simulink model "Model_SinglePhase_TwoArm"  (R2022a)
settings: Solver=VariableStepAuto  StartTime=0.0  StopTime=10.0  RelTol=1e-3
libraries: fl_lib x15
settings Model: Creator=chack  LastModifiedBy=chack

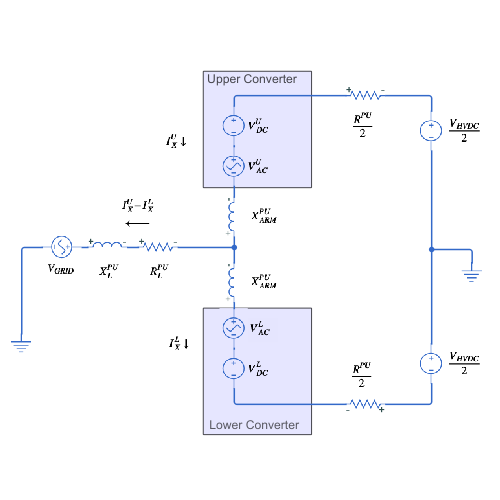
[thumbnail: Simulink's stored preview of the top-level diagram]
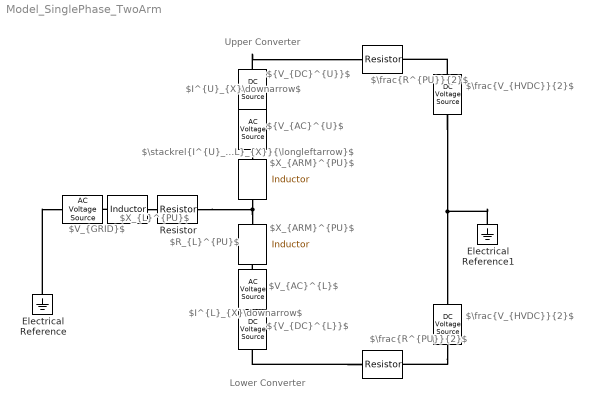
== system Model_SinglePhase_TwoArm ==
  note: $I^{U}_{X}\downarrow$
  note: Lower Converter
  note: Upper Converter
  note: ${V_{DC}^{U}}$
  note: $V_{GRID}$
  note: $R_{L}^{PU}$
  note: $X_{L}^{PU}$
  note: $\frac{V_{HVDC}}{2}$
  note: $\frac{V_{HVDC}}{2}$
  note: $\frac{R^{PU}}{2}$
  note: ${V_{AC}^{U}$
  note: $X_{ARM}^{PU}$
  note: ${V_{DC}^{L}}$
  note: $V_{AC}^{L}$
  note: $X_{ARM}^{PU}$
  note: $\frac{R^{PU}}{2}$
  note: $\stackrel{I^{U}_{X}-I^{L}_{X}}{\longleftarrow}$
  note: $I^{L}_{X}\downarrow$
  " " : fl_lib/Electrical/Electrical Sources/AC Voltage Source  amp=1 V  shift=0 deg  frequency=60 Hz  omega=0 rad/s
      settings: SourceProductBaseCode=PW,SS,VE
  "  " : fl_lib/Electrical/Electrical Elements/Inductor  l=1e-6 H  r=0 Ohm  g=1e-9 1/Ohm  i_specify=off  i_priority=None  i=0 A  i_nominal_specify=off  i_nominal_unit=A  i_nominal_value=1  v_specify=off  v_priority=None  v=0 V  v_nominal_specify=off  v_nominal_unit=V  v_nominal_value=1  i_L_specify=off  i_L_priority=High  i_L=0 A  i_L_nominal_specify=off  i_L_nominal_unit=A  i_L_nominal_value=1
      settings: SourceProductBaseCode=PW,SS,VE
  "   " : fl_lib/Electrical/Electrical Elements/Inductor  l=1e-6 H  r=0 Ohm  g=1e-9 1/Ohm  i_specify=off  i_priority=None  i=0 A  i_nominal_specify=off  i_nominal_unit=A  i_nominal_value=1  v_specify=off  v_priority=None  v=0 V  v_nominal_specify=off  v_nominal_unit=V  v_nominal_value=1  i_L_specify=off  i_L_priority=High  i_L=0 A  i_L_nominal_specify=off  i_L_nominal_unit=A  i_L_nominal_value=1
      settings: SourceProductBaseCode=PW,SS,VE
  "    " : fl_lib/Electrical/Electrical Sources/DC Voltage Source  v0=1 V
      settings: SourceProductBaseCode=PW,SS,VE
  "     " : fl_lib/Electrical/Electrical Sources/DC Voltage Source  v0=1 V
      settings: SourceProductBaseCode=PW,SS,VE
  "       " : fl_lib/Electrical/Electrical Elements/Resistor  R=1 Ohm  i_specify=off  i_priority=None  i=0 A  i_nominal_specify=off  i_nominal_unit=A  i_nominal_value=1  v_specify=off  v_priority=None  v=0 V  v_nominal_specify=off  v_nominal_unit=V  v_nominal_value=1
      settings: SourceProductBaseCode=PW,SS,VE
  "         " : fl_lib/Electrical/Electrical Elements/Resistor  R=1 Ohm  i_specify=off  i_priority=None  i=0 A  i_nominal_specify=off  i_nominal_unit=A  i_nominal_value=1  v_specify=off  v_priority=None  v=0 V  v_nominal_specify=off  v_nominal_unit=V  v_nominal_value=1
      settings: SourceProductBaseCode=PW,SS,VE
  "            " : fl_lib/Electrical/Electrical Sources/AC Voltage Source  amp=1 V  shift=0 deg  frequency=60 Hz  omega=0 rad/s
      settings: SourceProductBaseCode=PW,SS,VE
  "                " : fl_lib/Electrical/Electrical Sources/DC Voltage Source  v0=1 V
      settings: SourceProductBaseCode=PW,SS,VE
  "                             " : fl_lib/Electrical/Electrical Sources/DC Voltage Source  v0=1 V
      settings: SourceProductBaseCode=PW,SS,VE
  "                                 " : fl_lib/Electrical/Electrical Sources/AC Voltage Source  amp=1 V  shift=0 deg  frequency=60 Hz  omega=0 rad/s
      settings: SourceProductBaseCode=PW,SS,VE
  "                                                    " : fl_lib/Electrical/Electrical Elements/Inductor  l=1e-6 H  r=0 Ohm  g=1e-9 1/Ohm  i_specify=off  i_priority=None  i=0 A  i_nominal_specify=off  i_nominal_unit=A  i_nominal_value=1  v_specify=off  v_priority=None  v=0 V  v_nominal_specify=off  v_nominal_unit=V  v_nominal_value=1  i_L_specify=off  i_L_priority=High  i_L=0 A  i_L_nominal_specify=off  i_L_nominal_unit=A  i_L_nominal_value=1
      settings: SourceProductBaseCode=PW,SS,VE
  Electrical Reference : fl_lib/Electrical/Electrical Elements/Electrical Reference
      settings: SourceProductBaseCode=PW,SS,VE
  Electrical Reference1 : fl_lib/Electrical/Electrical Elements/Electrical Reference
      settings: SourceProductBaseCode=PW,SS,VE
  Resistor : fl_lib/Electrical/Electrical Elements/Resistor  R=1 Ohm  i_specify=off  i_priority=None  i=0 A  i_nominal_specify=off  i_nominal_unit=A  i_nominal_value=1  v_specify=off  v_priority=None  v=0 V  v_nominal_specify=off  v_nominal_unit=V  v_nominal_value=1
      settings: SourceProductBaseCode=PW,SS,VE
  connections:
  "            "/LConn1 -- "                "/RConn1
  "     "/RConn1 -- Electrical Reference1/LConn1 -- "    "/LConn1
  "                "/LConn1 -- "       "/LConn1
  "  "/LConn1 -- " "/LConn1
  Electrical Reference/LConn1 -- " "/RConn1
  "  "/RConn1 -- Resistor/LConn1
  "            "/RConn1 -- "   "/RConn1
  Resistor/RConn1 -- "   "/LConn1 -- "                                                    "/RConn1
  "         "/RConn1 -- "                             "/RConn1
  "                                 "/LConn1 -- "                                                    "/LConn1
  "                             "/LConn1 -- "                                 "/RConn1
  "     "/LConn1 -- "       "/RConn1
  "    "/RConn1 -- "         "/LConn1
